simulink model "asbCubeSatVehicleOperator"  (R2022a)
settings: Solver=VariableStepAuto  StartTime=0.0  StopTime=10.0  RelTol=1e-3
undefined symbols (not defined in the file): CubeSatTimeStep
libraries: simulink x1
settings Model: DataDictionary=asbCubeSatArchInterfaceData.sldd  Creator=The MathWorks, Inc.  LastModifiedBy=4jack
settings SolverCC: AlgebraicLoopSolver=TrustRegion  MaxZcPerStep=1
settings DebuggingCC: UnconnectedInputMsg=warning  UnconnectedOutputMsg=warning  UnconnectedLineMsg=warning  SFMachineParentedDataDiag=warning
settings RTWCC: DLArmComputeVersion=19.05

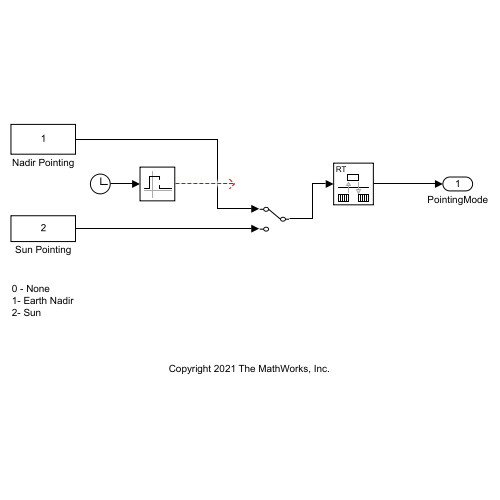
[thumbnail: Simulink's stored preview of the top-level diagram]
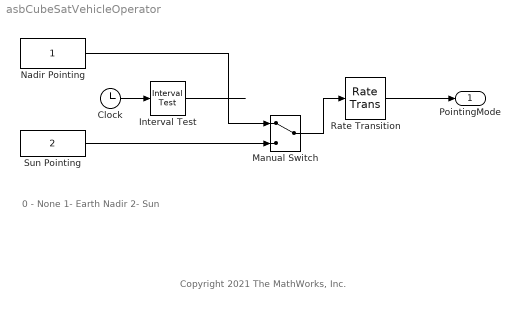
== system asbCubeSatVehicleOperator ==
  note: Copyright 2021 The MathWorks, Inc.
  note: 0 - None
      | 1- Earth Nadir
      | 2- Sun
  Clock : Clock
  Interval Test : simulink/Logic and Bit Operations/Interval Test  IntervalClosedRight=off  uplimit=10000000  IntervalClosedLeft=on  lowlimit=0  OutDataTypeStr=boolean
  Manual Switch : ManualSwitch
  Nadir Pointing : Constant  SampleTime=CubeSatTimeStep
  Rate Transition : RateTransition  OutPortSampleTime=CubeSatTimeStep
  Sun Pointing : Constant  Value=2  SampleTime=CubeSatTimeStep
  PointingMode : Outport
  wires:
  Clock/1 -> Interval Test/1
  Interval Test/1 -> ?
  Nadir Pointing/1 -> Manual Switch/1
  Sun Pointing/1 -> Manual Switch/2
  Manual Switch/1 -> Rate Transition/1
  Rate Transition/1 -> PointingMode/1
